simulink model "Examen_parte1"  (R2013a)
settings: Solver=ode45  StartTime=0.0  StopTime=10  RelTol=1e-3
settings Model: Creator=Miguel  LastModifiedBy=Miguel

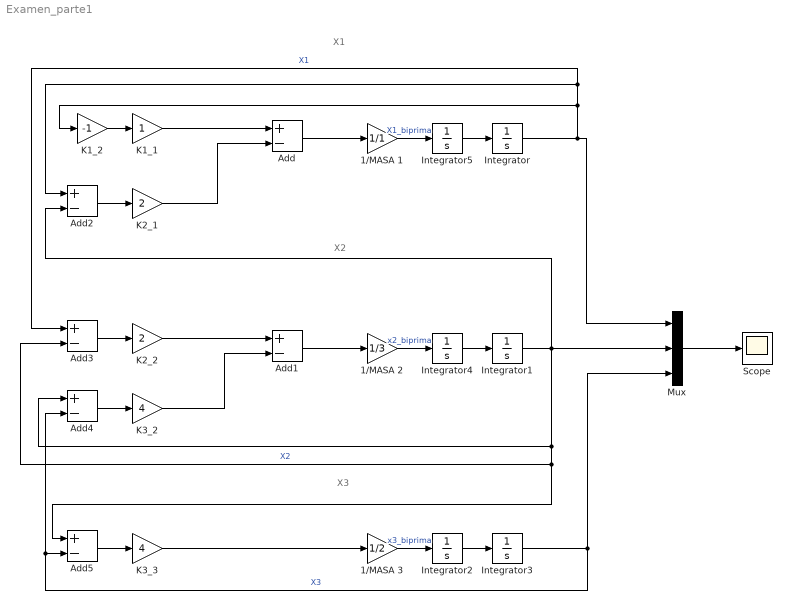
== system Examen_parte1 ==
  note: X1
  note: X3
  note: X2
  1/MASA 1 : Gain  Gain=1/1
  1/MASA 2 : Gain  Gain=1/3
  1/MASA 3 : Gain  Gain=1/2
  Add{,1..5} (6 alike) : Sum  Inputs=+-
  Integrator{,1..4} (5 alike) : Integrator
  Integrator5 : Integrator  InitialCondition=1
  K1_1 : Gain
  K1_2 : Gain  Gain=-1
  K2_1 : Gain  Gain=2
  K2_2 : Gain  Gain=2
  K3_2 : Gain  Gain=4
  K3_3 : Gain  Gain=4
  Mux : Mux  Inputs=3
  Scope : Scope
      settings: ShowLegends=on
  wires:
  Add/1 -> 1/MASA 1/1
  Add1/1 -> 1/MASA 2/1
  Add2/1 -> K2_1/1
  Add3/1 -> K2_2/1
  Add4/1 -> K3_2/1
  1/MASA 1/1 -> Integrator5/1  "X1_biprima"
  1/MASA 2/1 -> Integrator4/1  "x2_biprima"
  1/MASA 3/1 -> Integrator2/1  "x3_biprima"
  Integrator/1 -> Add3/1, Add2/1, K1_2/1, Mux/1  "X1"
  Integrator1/1 -> Add5/1, Add3/2, Add4/1, Add2/2, Mux/2  "X2"
  Integrator2/1 -> Integrator3/1
  Mux/1 -> Scope/1
  Add5/1 -> K3_3/1
  K3_3/1 -> 1/MASA 3/1
  Integrator3/1 -> Mux/3, Add4/2, Add5/2  "X3"
  Integrator4/1 -> Integrator1/1
  Integrator5/1 -> Integrator/1
  K2_2/1 -> Add1/1
  K3_2/1 -> Add1/2
  K2_1/1 -> Add/2
  K1_1/1 -> Add/1
  K1_2/1 -> K1_1/1
